simulink model "test_origin"  (R2024b)
settings: Solver=VariableStepAuto  StartTime=0.0  StopTime=2  RelTol=1e-3
values from neighbouring files (symbols this model uses):
  B = zeros(img_h, img_w)    [code_params.m]
  eye_mat = eye(3)    [code_params.m]
  K = [fx, s, cx ... (first row only)    [code_params.m]
  mesh_data =     [triangle_mesh_bus.mat]
  texture_map = zeros(texture_resol,texture_resol)    [code_params.m]
undefined symbols (not defined in the file or in its folder): camera0, duration, light_model, light_source, link, link_name, model_name, world_pose
libraries: robotgazebolib x10, robotcorelib x2
(part 1 of 2)
settings Model: Creator=seunghyunpyo  LastModifiedBy=seunghyunpyo

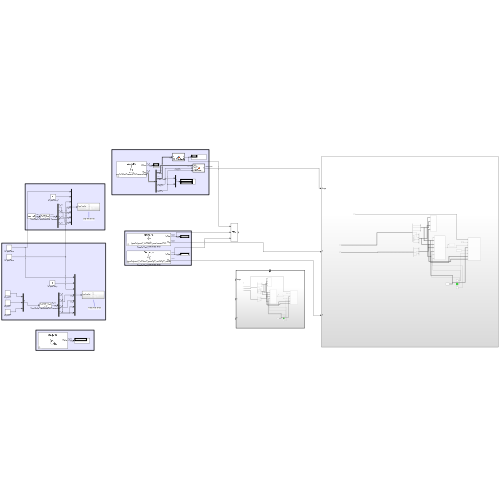
[thumbnail: Simulink's stored preview of the top-level diagram]
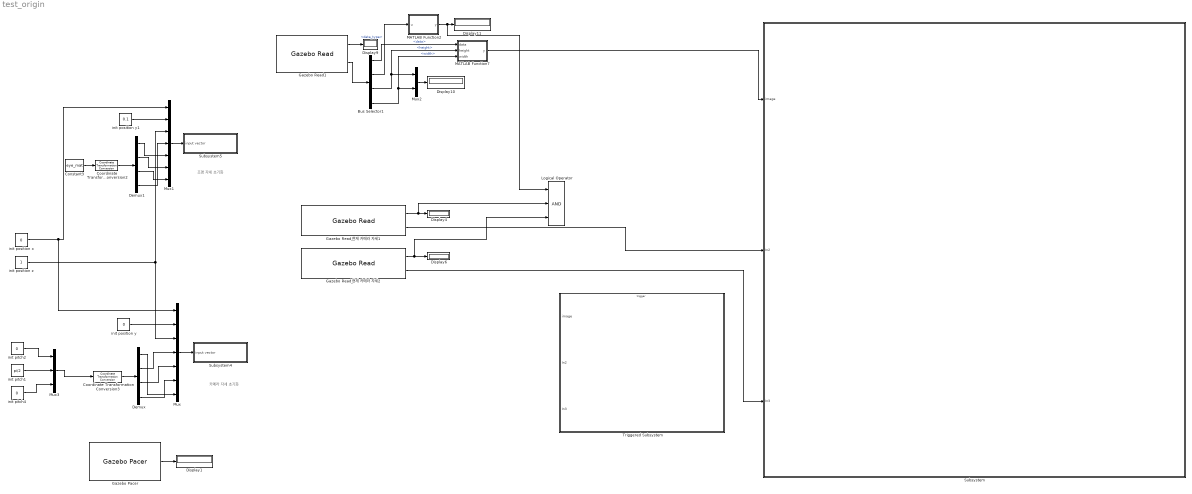
== system test_origin ==
  note: 카메라 자세 초기화
  note: 조명 자세 초기화
  Bus Selector1 : BusSelector  OutputSignals=data,data_type,height,width
  Constant3 : Constant  Value=eye_mat
  Coordinate Transformation Conversion2 : robotcorelib/Coordinate Transformation Conversion  InputRepresentation=Rotation Matrix  InputEulerSequence=ZYX  ShowTrVecInputPort=on  OutputRepresentation=Quaternion  OutputEulerSequence=XYZ  ShowTrVecOutputPort=on  SimulateUsing=Interpreted execution
  Coordinate Transformation Conversion3 : robotcorelib/Coordinate Transformation Conversion  InputRepresentation=Euler Angles  InputEulerSequence=XYZ  ShowTrVecInputPort=on  OutputRepresentation=Quaternion  OutputEulerSequence=XYZ  ShowTrVecOutputPort=on  SimulateUsing=Interpreted execution
  Demux : Demux
  Demux1 : Demux
  Display{1,4,6,9..11} (6 alike) : Display
  Gazebo Pacer : robotgazebolib/Gazebo Pacer  ResetBehavior=Reset Gazebo simulation time  SampleTime=0.01
  Gazebo Read1 : robotgazebolib/Gazebo Read  topicSource=From Gazebo  topic=/gazebo/default/camera0/link/camera/image  messageType=gazebo_msgs/Image  sampleTime=0.01  fixedAxisBusStatus=off  jointAxisCount=2
  Gazebo Read_현재 카메라 자세1 : robotgazebolib/Gazebo Read  topicSource=From Gazebo  topic=/gazebo/ground_truth/world_pose/camera0/link  messageType=gazebo_msgs/Pose  sampleTime=0.01  fixedAxisBusStatus=off  jointAxisCount=2
  Gazebo Read_현재 카메라 자세2 : robotgazebolib/Gazebo Read  topicSource=From Gazebo  topic=/gazebo/ground_truth/world_pose/light_model/light_source  messageType=gazebo_msgs/Pose  sampleTime=0.01  fixedAxisBusStatus=off  jointAxisCount=2
  Logical Operator : Logic  Inputs=3  AllPortsSameDT=off  OutDataTypeStr=boolean
  MATLAB Function2 : MATLAB Function  TreatAsAtomicUnit=on
  MATLAB Function7 : MATLAB Function  TreatAsAtomicUnit=on
  Mux : Mux  Inputs=7
  Mux1 : Mux  Inputs=7
  Mux2 : Mux  Inputs=2
  Mux3 : Mux  Inputs=3
  Subsystem : Subsystem
  Subsystem4 : Subsystem
  Subsystem5 : Subsystem
  Triggered Subsystem : Subsystem  TreatAsAtomicUnit=on
  init pitch1 : Constant  Value=pi/2
  init pitch2 : Constant  Value=0
  init pitch4 : Constant  Value=0
  init position x : Constant  Value=0
  init position y : Constant  Value=0
  init position y1 : Constant  Value=0.1
  init position z : Constant
  wires:
  Coordinate Transformation Conversion3/1 -> Demux/1
  Demux1/3 -> Mux1/7
  Mux3/1 -> Coordinate Transformation Conversion3/1
  Demux/1 -> Mux/7
  init pitch4/1 -> Mux3/3
  init pitch2/1 -> Mux3/1
  Mux/1 -> Subsystem4/1(input vector)
  Gazebo Read1/2 -> Bus Selector1/1
  Mux2/1 -> Display10/1
  Constant3/1 -> Coordinate Transformation Conversion2/1
  init position y1/1 -> Mux1/2
  Demux/4 -> Mux/6
  Demux/3 -> Mux/5
  init position y/1 -> Mux/2
  Gazebo Pacer/1 -> Display1/1
  init position z/1 -> Mux/3, Mux1/3
  Demux/2 -> Mux/4
  init position x/1 -> Mux/1, Mux1/1
  MATLAB Function2/1(y) -> Logical Operator/1, Display11/1
  Bus Selector1/4 -> MATLAB Function7/3(width), Mux2/2  "<width>"
  Bus Selector1/2 -> MATLAB Function2/1(u)  "<data_type>"
  init pitch1/1 -> Mux3/2
  Gazebo Read1/1 -> Display9/1
  Demux1/1 -> Mux1/5
  Bus Selector1/3 -> MATLAB Function7/2(height), Mux2/1  "<height>"
  Mux1/1 -> Subsystem5/1(input vector)
  Demux1/4 -> Mux1/4
  Demux1/2 -> Mux1/6
  Bus Selector1/1 -> MATLAB Function7/1(data)  "<data>"
  Coordinate Transformation Conversion2/1 -> Demux1/1
  Gazebo Read_현재 카메라 자세2/1 -> Logical Operator/3, Display6/1
  Gazebo Read_현재 카메라 자세1/1 -> Logical Operator/2, Display4/1
  MATLAB Function7/1(y) -> Subsystem/1(image)
  Gazebo Read_현재 카메라 자세1/2 -> Subsystem/2(In2)
  Gazebo Read_현재 카메라 자세2/2 -> Subsystem/3(In3)

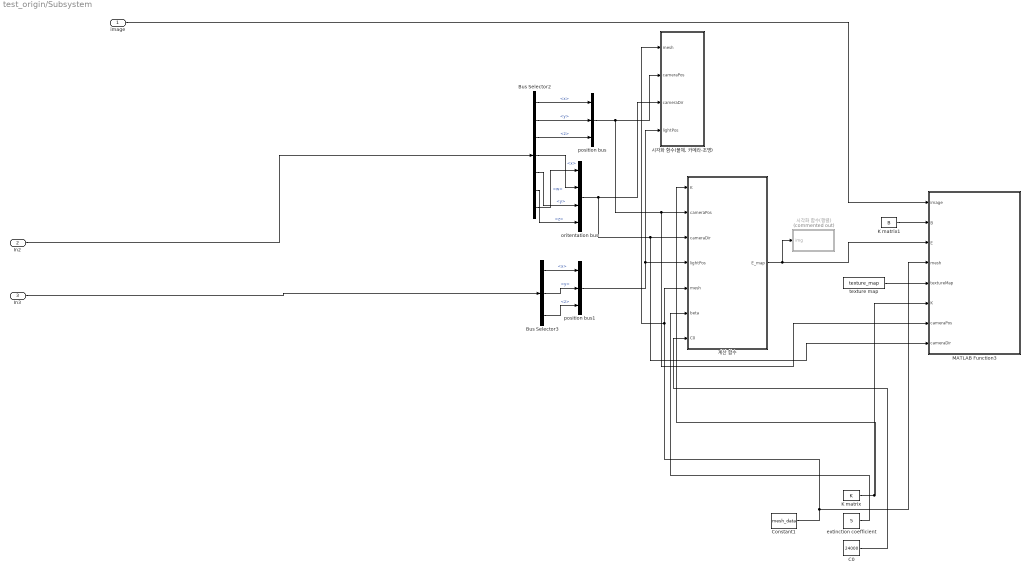
== system test_origin/Subsystem ==
  image : Inport
  In2 : Inport  Port=2
  In3 : Inport  Port=3
  Bus Selector2 : BusSelector  OutputSignals=position.x,position.y,position.z,orientation.x,orientation.y,orientation.z,orientation.w
  Bus Selector3 : BusSelector  OutputSignals=position.x,position.y,position.z
  C0 : Constant  Value=24000
  Constant1 : Constant  Value=mesh_data  OutDataTypeStr=Bus: slBus1
  K matrix : Constant  Value=K
  K matrix1 : Constant  Value=B
  MATLAB Function3 : MATLAB Function  TreatAsAtomicUnit=on
  extinction coefficient : Constant  Value=5
  oritentation bus : BusCreator  Inputs=4
  position bus : BusCreator  Inputs=3
  position bus1 : BusCreator  Inputs=3
  texture map : Constant  Value=texture_map
  계산 함수 : MATLAB Function  TreatAsAtomicUnit=on
  "시각화 함수(물체, 카메라-조명)" : MATLAB Function  TreatAsAtomicUnit=on
  시각화 함수(행렬) : MATLAB Function  Commented=on  TreatAsAtomicUnit=on
  wires:
  In3/1 -> Bus Selector3/1
  image/1 -> MATLAB Function3/1(image)
  Bus Selector2/6 -> oritentation bus/4  "<z>"
  In2/1 -> Bus Selector2/1
  Bus Selector2/4 -> oritentation bus/2  "<x>"
  oritentation bus/1 -> MATLAB Function3/8(cameraDir), 계산 함수/3(cameraDir), "시각화 함수(물체, 카메라-조명)"/3(cameraDir)
  position bus/1 -> MATLAB Function3/7(cameraPos), 계산 함수/2(cameraPos), "시각화 함수(물체, 카메라-조명)"/2(cameraPos)
  Bus Selector3/1 -> position bus1/1  "<x>"
  Bus Selector2/1 -> position bus/1  "<x>"
  Bus Selector2/3 -> position bus/3  "<z>"
  Bus Selector3/2 -> position bus1/2  "<y>"
  Bus Selector3/3 -> position bus1/3  "<z>"
  Bus Selector2/2 -> position bus/2  "<y>"
  position bus1/1 -> 계산 함수/4(lightPos), "시각화 함수(물체, 카메라-조명)"/4(lightPos)
  C0/1 -> 계산 함수/7(C0)
  Bus Selector2/5 -> oritentation bus/3  "<y>"
  texture map/1 -> MATLAB Function3/5(textureMap)
  Bus Selector2/7 -> oritentation bus/1  "<w>"
  K matrix1/1 -> MATLAB Function3/2(B)
  Constant1/1 -> MATLAB Function3/4(mesh), "시각화 함수(물체, 카메라-조명)"/1(mesh), 계산 함수/5(mesh)
  K matrix/1 -> MATLAB Function3/6(K), 계산 함수/1(K)
  계산 함수/1(E_map) -> 시각화 함수(행렬)/1(img), MATLAB Function3/3(E)
  extinction coefficient/1 -> 계산 함수/6(beta)

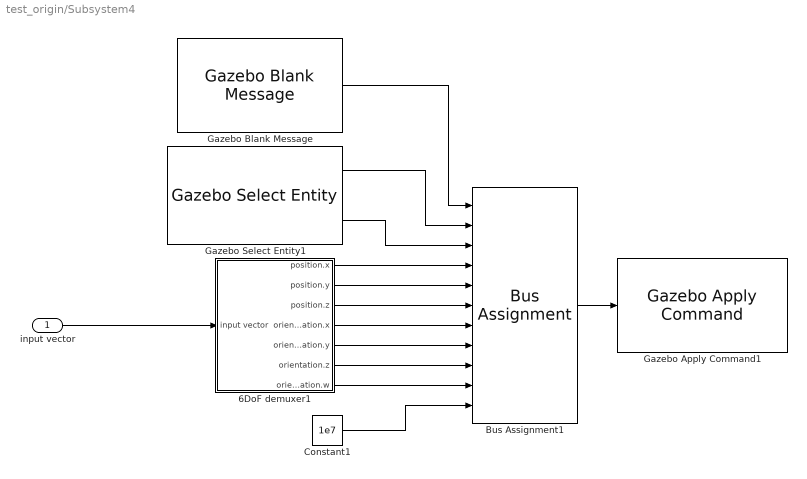
== system test_origin/Subsystem4 ==
  input vector : Inport
  6DoF demuxer1 : Subsystem
  Bus Assignment1 : BusAssignment  AssignedSignals=model_name,link_name,world_pose.position.x,world_pose.position.y,world_pose.position.z,world_pose.orientation.x,world_pose.orientation.y,world_pose.orientation.z,world_pose.orientation.w,duration.nano_seconds
  Constant1 : Constant  Value=1e7
  Gazebo Apply Command1 : robotgazebolib/Gazebo Apply Command  cmdType=SetLinkWorldPose  sampleTime=0.01
  Gazebo Blank Message : robotgazebolib/Gazebo Blank Message  msgType=SetLinkWorldPose  sampleTime=0.01  busName='Gazebo_SL_Bus_gazebo_msgs_SetLinkWorldPose'
  Gazebo Select Entity1 : robotgazebolib/Gazebo Select Entity  modelElemName=camera0/link  outputArraySize=128  OutputLabel=Link  SelectType=Link
  wires:
  Constant1/1 -> Bus Assignment1/11
  6DoF demuxer1/1(position.x) -> Bus Assignment1/4
  6DoF demuxer1/2(position.y) -> Bus Assignment1/5
  input vector/1 -> 6DoF demuxer1/1(input vector)
  Bus Assignment1/1 -> Gazebo Apply Command1/1
  Gazebo Blank Message/1 -> Bus Assignment1/1
  6DoF demuxer1/6(orientation.z) -> Bus Assignment1/9
  6DoF demuxer1/3(position.z) -> Bus Assignment1/6
  6DoF demuxer1/5(orientation.y) -> Bus Assignment1/8
  6DoF demuxer1/4(orientation.x) -> Bus Assignment1/7
  Gazebo Select Entity1/2 -> Bus Assignment1/3
  Gazebo Select Entity1/1 -> Bus Assignment1/2
  6DoF demuxer1/7(orientation.w) -> Bus Assignment1/10

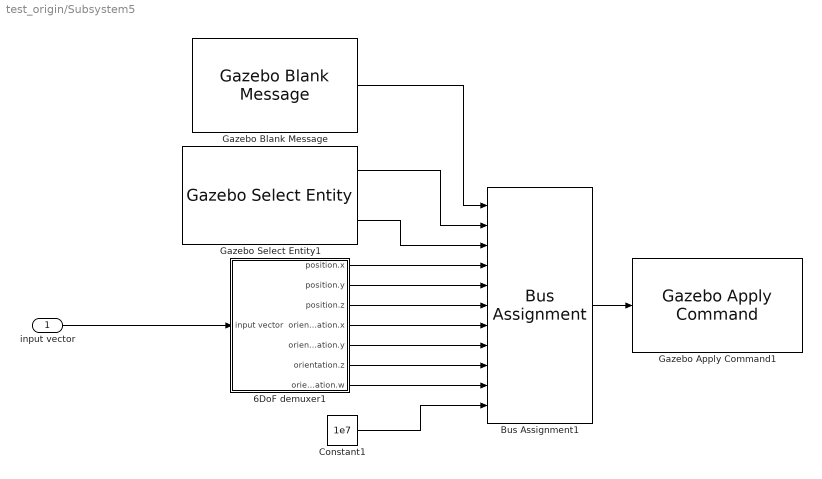
== system test_origin/Subsystem5 ==
  input vector : Inport
  6DoF demuxer1 : Subsystem
  Bus Assignment1 : BusAssignment  AssignedSignals=model_name,link_name,world_pose.position.x,world_pose.position.y,world_pose.position.z,world_pose.orientation.x,world_pose.orientation.y,world_pose.orientation.z,world_pose.orientation.w,duration.nano_seconds
  Constant1 : Constant  Value=1e7
  Gazebo Apply Command1 : robotgazebolib/Gazebo Apply Command  cmdType=SetLinkWorldPose  sampleTime=0.01
  Gazebo Blank Message : robotgazebolib/Gazebo Blank Message  msgType=SetLinkWorldPose  sampleTime=0.01  busName='Gazebo_SL_Bus_gazebo_msgs_SetLinkWorldPose'
  Gazebo Select Entity1 : robotgazebolib/Gazebo Select Entity  modelElemName=light_model/light_source  outputArraySize=128  OutputLabel=Link  SelectType=Link
  wires:
  6DoF demuxer1/7(orientation.w) -> Bus Assignment1/10
  Gazebo Select Entity1/1 -> Bus Assignment1/2
  Gazebo Select Entity1/2 -> Bus Assignment1/3
  6DoF demuxer1/4(orientation.x) -> Bus Assignment1/7
  6DoF demuxer1/5(orientation.y) -> Bus Assignment1/8
  6DoF demuxer1/3(position.z) -> Bus Assignment1/6
  6DoF demuxer1/6(orientation.z) -> Bus Assignment1/9
  Gazebo Blank Message/1 -> Bus Assignment1/1
  Bus Assignment1/1 -> Gazebo Apply Command1/1
  6DoF demuxer1/2(position.y) -> Bus Assignment1/5
  6DoF demuxer1/1(position.x) -> Bus Assignment1/4
  Constant1/1 -> Bus Assignment1/11
  input vector/1 -> 6DoF demuxer1/1(input vector)

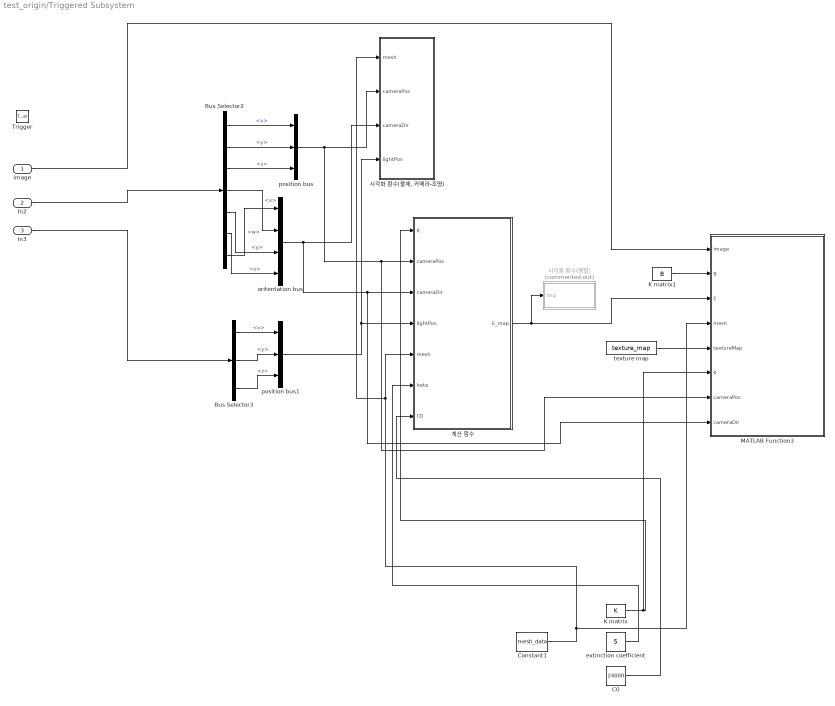
== system test_origin/Triggered Subsystem ==
  image : Inport
  In2 : Inport  Port=2
  In3 : Inport  Port=3
  Trigger : TriggerPort  VariantControl=(inherit)
  Bus Selector2 : BusSelector  OutputSignals=position.x,position.y,position.z,orientation.x,orientation.y,orientation.z,orientation.w
  Bus Selector3 : BusSelector  OutputSignals=position.x,position.y,position.z
  C0 : Constant  Value=24000
  Constant1 : Constant  Value=mesh_data  OutDataTypeStr=Bus: slBus1
  K matrix : Constant  Value=K
  K matrix1 : Constant  Value=B
  MATLAB Function3 : MATLAB Function  TreatAsAtomicUnit=on
  extinction coefficient : Constant  Value=5
  oritentation bus : BusCreator  Inputs=4
  position bus : BusCreator  Inputs=3
  position bus1 : BusCreator  Inputs=3
  texture map : Constant  Value=texture_map
  계산 함수 : MATLAB Function  TreatAsAtomicUnit=on
  "시각화 함수(물체, 카메라-조명)" : MATLAB Function  TreatAsAtomicUnit=on
  시각화 함수(행렬) : MATLAB Function  Commented=on  TreatAsAtomicUnit=on
  wires:
  image/1 -> MATLAB Function3/1(image)
  Bus Selector2/6 -> oritentation bus/4  "<z>"
  In3/1 -> Bus Selector3/1
  In2/1 -> Bus Selector2/1
  계산 함수/1(E_map) -> 시각화 함수(행렬)/1(img), MATLAB Function3/3(E)
  K matrix/1 -> MATLAB Function3/6(K), 계산 함수/1(K)
  Constant1/1 -> MATLAB Function3/4(mesh), "시각화 함수(물체, 카메라-조명)"/1(mesh), 계산 함수/5(mesh)
  position bus1/1 -> 계산 함수/4(lightPos), "시각화 함수(물체, 카메라-조명)"/4(lightPos)
  Bus Selector2/4 -> oritentation bus/2  "<x>"
  texture map/1 -> MATLAB Function3/5(textureMap)
  extinction coefficient/1 -> 계산 함수/6(beta)
  position bus/1 -> MATLAB Function3/7(cameraPos), 계산 함수/2(cameraPos), "시각화 함수(물체, 카메라-조명)"/2(cameraPos)
  Bus Selector3/3 -> position bus1/3  "<z>"
  Bus Selector2/2 -> position bus/2  "<y>"
  C0/1 -> 계산 함수/7(C0)
  Bus Selector3/2 -> position bus1/2  "<y>"
  oritentation bus/1 -> MATLAB Function3/8(cameraDir), 계산 함수/3(cameraDir), "시각화 함수(물체, 카메라-조명)"/3(cameraDir)
  Bus Selector2/3 -> position bus/3  "<z>"
  Bus Selector3/1 -> position bus1/1  "<x>"
  K matrix1/1 -> MATLAB Function3/2(B)
  Bus Selector2/5 -> oritentation bus/3  "<y>"
  Bus Selector2/7 -> oritentation bus/1  "<w>"
  Bus Selector2/1 -> position bus/1  "<x>"

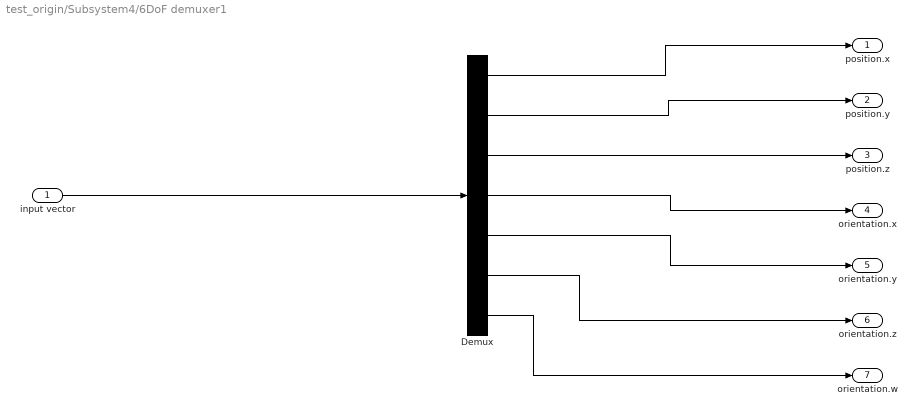
== system test_origin/Subsystem4/6DoF demuxer1 ==
  input vector : Inport
  Demux : Demux  Outputs=7
  position.x : Outport
  position.y : Outport  Port=2
  position.z : Outport  Port=3
  orientation.x : Outport  Port=4
  orientation.y : Outport  Port=5
  orientation.z : Outport  Port=6
  orientation.w : Outport  Port=7
  wires:
  input vector/1 -> Demux/1
  Demux/1 -> position.x/1
  Demux/2 -> position.y/1
  Demux/3 -> position.z/1
  Demux/4 -> orientation.x/1
  Demux/5 -> orientation.y/1
  Demux/6 -> orientation.z/1
  Demux/7 -> orientation.w/1

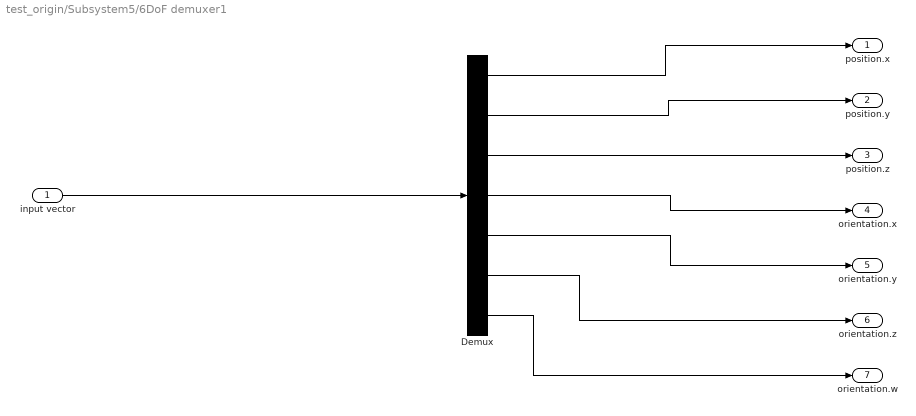
== system test_origin/Subsystem5/6DoF demuxer1 ==
  input vector : Inport
  Demux : Demux  Outputs=7
  position.x : Outport
  position.y : Outport  Port=2
  position.z : Outport  Port=3
  orientation.x : Outport  Port=4
  orientation.y : Outport  Port=5
  orientation.z : Outport  Port=6
  orientation.w : Outport  Port=7
  wires:
  Demux/7 -> orientation.w/1
  Demux/6 -> orientation.z/1
  Demux/5 -> orientation.y/1
  Demux/4 -> orientation.x/1
  Demux/3 -> position.z/1
  Demux/2 -> position.y/1
  Demux/1 -> position.x/1
  input vector/1 -> Demux/1

== matlab function test_origin/MATLAB Function7 ==
  data: data input; height input; width input; y output [..255]
function y  = plotImage(data, height, width)

coder.extrinsic('imshow');
coder.extrinsic('helperPlotImage');

persistent h

if isempty(h)
    h = newplot(figure());
end


y = zeros(height, width, 3, 'uint8');
if ~isempty(data) && ~isscalar(data)
    y(:) = helperPlotImage(data, height, width);
end
imshow(y, 'Parent', h);

== matlab function test_origin/Subsystem/시각화 함수(물체, 카메라-조명) ==
  data: mesh input; cameraPos input; cameraDir input; lightPos input
function viz_scene(mesh, cameraPos, cameraDir, lightPos)

    persistent figHandle; % Figure 핸들을 저장할 persistent 변수

    if isempty(figHandle)
        % Figure가 없으면 (처음 실행) figHandle 초기화
        figHandle = figure;
        set(figHandle, 'Name', 'Scene Visualization'); % (선택 사항) 창 제목 설정
    elseif ~ishandle(figHandle) || ~strcmp(get(figHandle, 'Type'), 'figure')
        % Figure 핸들이 유효하지 않으면 (Figure가 닫힌 경우)
        figHandle = figure; % 새 Figure 생성
        set(figHandle, 'Name', 'Scene Visualization');
    end
    
    figure(figHandle); % 해당 Figure를 활성화
    clf;    % Figure 내용 clear  % clf(figHandle) 대신 clf 사용

    faces_vertex = mesh.faces.v;
    vertices = mesh.vertices;
    quat_link_world = quaternion(cameraDir(1), cameraDir(2), cameraDir(3), cameraDir(4));
    R_w2link = rotmat(quat_link_world, 'frame');         % 월드 -> 링크 좌표계 회전
    R_link2cam =[0 -1 0; 0 0 -1; 1 0 0];                % 링크 좌표계 -> 카메라 좌표계 회전


    % 1. 메쉬 그리기
    subplot(1, 2, 1); % 이 부분은 그대로 유지
    trisurf(faces_vertex, vertices(:,1), vertices(:,2), vertices(:,3), 'FaceColor', 'cyan', 'EdgeColor', 'k');
    hold on;
    % Face 중앙에 Face 번호 표시
    for i = 1:int32(size(faces_vertex, 1))
        % 현재 Face의 정점 3개 가져오기
        face_vertices = vertices(faces_vertex(i, :), :);

        % Face의 중심 좌표 계산
        face_center = mean(face_vertices, 1);

        % Face의 중앙에 번호 표시
        text(face_center(1), face_center(2), face_center(3), sprintf('%d',i), ...
            'FontSize', 12, 'FontWeight', 'bold', 'Color', 'r');
    end

    % 2. 카메라 위치 및 방향 (월드 좌표계)
    cameraPos_world = cameraPos; % 월드 좌표계에서의 카메라 위치
    R_world_to_cam = R_link2cam * R_w2link; % 카메라 방향 변환 행렬
    % 카메라 X축 (빨강)
    quiver3(cameraPos_world(1), cameraPos_world(2), cameraPos_world(3), ...
        R_world_to_cam(1,1), R_world_to_cam(2,1), R_world_to_cam(3,1), 0.3, 'r', 'LineWidth', 2, 'MaxHeadSize', 0.5);
    % 카메라 Y축 (초록)
    quiver3(cameraPos_world(1), cameraPos_world(2), cameraPos_world(3), ...
        R_world_to_cam(1,2), R_world_to_cam(2,2), R_world_to_cam(3,2), 0.3, 'g', 'LineWidth', 2, 'MaxHeadSize', 0.5);
    % 카메라 Z축 (파랑)
    quiver3(cameraPos_world(1), cameraPos_world(2), cameraPos_world(3), ...
        R_world_to_cam(1,3), R_world_to_cam(2,3), R_world_to_cam(3,3), 0.3, 'b', 'LineWidth', 2, 'MaxHeadSize', 0.5);

    % 카메라 위치 (빨간색 점)
    plot3(cameraPos_world(1), cameraPos_world(2), cameraPos_world(3), 'ro', 'MarkerSize', 8, 'MarkerFaceColor', 'r');
    % 3. 광원 위치
    plot3(lightPos(1), lightPos(2), lightPos(3), 'yo', 'MarkerSize', 10, 'MarkerFaceColor', 'y'); % 노란색 점
    % 축 및 레이블
    xlabel('X (World)');
    ylabel('Y (World)');
    zlabel('Z (World)');
    title('World Coordinate System (Mesh, Camera, Light)');
    axis equal;
    grid on;
    view(3);
    hold off;
end

== matlab function test_origin/Subsystem/시각화 함수(행렬) ==
  data: img input
function viz_mat(img)
    figure;
    imagesc(img);
    colorbar;
    title('E\_map (Scattering Lighting)');
    xlabel('Pixel X');
    ylabel('Pixel Y');
    axis image; % x, y 축 비율을 데이터에 맞게
end

== matlab function test_origin/Subsystem/계산 함수 ==
  data: K input; cameraPos input; cameraDir input; lightPos input; mesh input; beta input; C0 input; E_map output
function E_map = computeScatteringLighting(K, cameraPos, cameraDir, lightPos, mesh, beta, C0)
    % 입력:
    %   K: 3x3 Intrinsic Matrix (카메라 내부 파라미터 행렬)
    %   R_link: 3x3 Rotation Matrix (월드 좌표계 -> 링크 좌표계 회전 행렬)
    %   T: 3x1 Translation Vector (월드 좌표계 -> 링크 좌표계 이동 벡터)
    %   lightPos: 1x3 광원 위치 (월드 좌표계)
    %   mesh: 메쉬 데이터 (구조체)
    %       mesh.v:  정점(Vertices) 좌표 (Nx3 행렬, N: 정점 개수)
    %       mesh.f.v: 면(Faces)을 구성하는 정점 인덱스 (Mx3 행렬, M: 면 개수)
    %       mesh.f.vn: 면의 법선 벡터 (Mx3 행렬)
    %   beta: 감쇠 계수 (Attenuation Coefficient)
    %   C0: 광원의 초기 강도 (Initial Light Intensity)
    imageHeight = 480;
    imageWidth = 640;

    % 출력:
    %   E_map: imageHeight x imageWidth 크기의 2D 이미지. 각 픽셀은 해당 위치에 도달하는 빛의 에너지(세기)를 나타냄.

    % 1. 메쉬 데이터 가져오기
    vertices = mesh.vertices;      % 정점 좌표
    faces_vertex = mesh.faces.v; % 면을 구성하는 정점 인덱스
    normals = mesh.faces.vn;    % 면의 법선 벡터

    % 2. 출력 맵 초기화
    E_map = zeros(imageHeight, imageWidth); % 출력 이미지를 0으로 초기화
    numFaces = size(faces_vertex, 1);     % 면의 개수

    % 3. 월드 좌표계 -> 카메라 좌표계 변환 행렬 계산
    T_link = cameraPos; % 나중에 전치 주의!!

    quat_link_world = quaternion(cameraDir(1), cameraDir(2), cameraDir(3), cameraDir(4));
    R_w2link = rotmat(quat_link_world, 'frame')         % 월드 -> 링크 좌표계 회전
    R_link2cam =[0 -1 0; 0 0 -1; 1 0 0];                % 링크 좌표계 -> 카메라 좌표계 회전 
    
    Proj_w2link = [R_w2link, -R_w2link*T_link; 0,0,0,1];        % 동차 변환 행렬 (월드 -> 링크)
    Proj_link2Cam = [R_link2cam, zeros(3,1); zeros(1,3), 1];    % 동차 변환 행렬 (링크 -> 카메라)
    Proj_w2cam = Proj_link2Cam * Proj_w2link;                   % 동차 변환 행렬 (월드 -> 카메라)

    % 4. 광원 위치를 카메라 좌표계로 변환 (동차 좌표계 사용)
    lightPos_hom = [lightPos; 1]; % 광원 위치를 동차 좌표로
    lightPosCam_hom = Proj_w2cam * lightPos_hom;
    lightPosCam = lightPosCam_hom(1:3); % 다시 3차원 좌표로
    
   % 5. 각 면에 대해 반복
    for i = 1:numFaces
        % 5.1. 면의 세 정점 좌표 (월드 좌표계)
        v1 = vertices(faces_vertex(i, 1), :); % 첫 번째 정점
        v2 = vertices(faces_vertex(i, 2), :); % 두 번째 정점
        v3 = vertices(faces_vertex(i, 3), :); % 세 번째 정점

        % 5.2. 면 중심 (월드 좌표계)
        faceCenter = (v1 + v2 + v3) / 3;

        % 5.3. 면의 법선 벡터 (월드 좌표계, 정규화)
        normal = normals(i, :);
        normal = normal / norm(normal);

        % 5.4. 카메라 좌표계로 변환 (동차 좌표계 사용)
        faceCenter_hom = [faceCenter, 1]';
        faceCenterCam_hom = Proj_w2cam * faceCenter_hom;
        faceCenterCam = faceCenterCam_hom(1:3);

        v1_hom = [v1, 1]';
        v1_cam_hom = Proj_w2cam * v1_hom;
        v1_cam = v1_cam_hom(1:3);

        v2_hom = [v2, 1]';
        v2_cam_hom = Proj_w2cam * v2_hom;
        v2_cam = v2_cam_hom(1:3);

        v3_hom = [v3, 1]';
        v3_cam_hom = Proj_w2cam * v3_hom;
        v3_cam = v3_cam_hom(1:3);

        normal_hom = [normal, 0]'; % 방향 벡터는 마지막 요소가 0
        normalCam_hom = Proj_w2cam * normal_hom;
        normalCam = normalCam_hom(1:3);



        % 5.5. 광원 방향 (카메라 좌표계)
        lightDir = lightPosCam - faceCenterCam; % 면 중심 -> 광원
        lLS = norm(lightDir);              % 광원과 면 중심 사이의 거리
        lightDir = lightDir / lLS;           % 정규화

        % 5.6. Lambertian 반사 계수
        diffuseFactor = max(0, dot(normalCam, lightDir)); % (0 ~ 1)

        % 5.7. 직접광 (Ds) 계산
        Ds = (C0 * exp(-beta * lLS)) / (lLS^2);

        % 5.8. 산란 지점 (z) 계산 (카메라 좌표계)
        epsilon = 0.01; % 작은 값 (면에서 약간 떨어진 거리)
        z = faceCenterCam + epsilon * normalCam; % 면 중심에서 법선 방향으로

        % 5.9. 거리 계산 (카메라 좌표계)
        lLZ = norm(lightPosCam - z);     % 광원 -> 산란 지점
        lSZ = norm(z - faceCenterCam);   % 산란 지점 -> 면 중심
        lSC = norm(faceCenterCam);       % 면 중심 -> 카메라

        % 5.10. 산란광 (As) 계산
        As = (C0 * exp(-beta * (lLZ + lSZ))) / ((lLZ + lSZ)^2);

        % 5.11. 초기 조도, 최종 조도
        Es_initial = Ds + As;            % 직접광 + 산란광
        Es = Es_initial * exp(-beta * lSC); % 최종 감쇠

        % 5.12. 각 정점을 2D 이미지 좌표로 투영 (카메라 내부 파라미터 K 사용)
        v1_proj_hom = K * v1_cam;
        v1_proj = round(v1_proj_hom(1:2) / v1_proj_hom(3)); % 2D 픽셀 좌표

        v2_proj_hom = K * v2_cam;
        v2_proj = round(v2_proj_hom(1:2) / v2_proj_hom(3));

        v3_proj_hom = K * v3_cam;
        v3_proj = round(v3_proj_hom(1:2) / v3_proj_hom(3));


        % 5.13. 삼각형 래스터화 (Bresenham's Algorithm 기반)
        pixels = [];

        % 삼각형의 세 변을 따라 픽셀 좌표 생성
        pixels = [pixels; bresenham(v1_proj(1), v1_proj(2), v2_proj(1), v2_proj(2))];
        pixels = [pixels; bresenham(v2_proj(1), v2_proj(2), v3_proj(1), v3_proj(2))];
        pixels = [pixels; bresenham(v3_proj(1), v3_proj(2), v1_proj(1), v1_proj(2))];

        % 5.14. 삼각형 내부 픽셀에 대해 반복
        for p = 1:size(pixels, 1)
             x = pixels(p, 1); % 픽셀 x 좌표
             y = pixels(p, 2); % 픽셀 y 좌표

             % 픽셀이 이미지 범위 내에 있는지 확인
            if x < 1 || x > imageWidth || y < 1 || y > imageHeight
                continue;
            end

            % Barycentric Coordinates 계산
            [alpha, beta, gamma] = barycentric(x, y, v1_proj, v2_proj, v3_proj);

            if alpha >= 0 && beta >= 0 && gamma >= 0
                % 5.15. 픽셀 (x, y)에 E_s * diffuseFactor 값을 할당
                E_map(y, x) = Es * diffuseFactor;
            end
        end
    end % for i
end % function

% Bresenham's line algorithm 함수
function points = bresenham(x1, y1, x2, y2)
    % 입력: 두 점 (x1, y1), (x2, y2)
    % 출력: 두 점을 잇는 직선 상의 픽셀 좌표 (정수)

    points = [];
    dx = abs(x2 - x1);
    dy = abs(y2 - y1);
    sx = sign(x2 - x1);
    sy = sign(y2 - y1);
    err = dx - dy;

    x = x1;
    y = y1;

    while true
        points = [points; x, y];

        if x == x2 && y == y2
            break;
        end

        e2 = 2 * err;
        if e2 > -dy
            err = err - dy;
            x = x + sx;
        end
        if e2 < dx
            err = err + dx;
            y = y + sy;
        end
    end
end

% Barycentric coordinates 계산 함수
function [alpha, beta, gamma] = barycentric(x, y, v1, v2, v3)
    % 입력:
    %   x, y: 픽셀 좌표
    %   v1, v2, v3: 삼각형의 세 꼭지점 좌표 (2D)
    % 출력:
    %    alpha, beta, gamma: Barycentric Coordinates

    % 삼각형 면적 계산 (두 벡터의 외적)
    area = 0.5 * (-v2(2) * v3(1) + v1(2) * (-v2(1) + v3(1)) + v1(1) * (v2(2) - v3(2)) + v2(1) * v3(2));

    % 각 꼭지점에 대한 가중치 계산
    alpha = 0.5 * (-v2(2) * v3(1) + y * (-v2(1) + v3(1)) + x * (v2(2) - v3(2)) + v2(1) * v3(2)) / area;
    beta  = 0.5 * ( v1(2) * v3(1) - y * v3(1) + x * (-v1(2) + v3(2)) - v1(1) * v3(2)              ) / area;
    gamma = 0.5 * (-v1(2) * v2(1) + v1(2) * x + v2(2) * (-x + v1(1)) + y * (v2(1) - v1(1))) / area;

end

== matlab function test_origin/Triggered Subsystem/MATLAB Function3 ==
  data: image input; B input; E input; mesh input; textureMap input; K input; cameraPos input; cameraDir input
function processReflectance(image, B, E, mesh, textureMap, K, cameraPos, cameraDir)

    image = double(image);
    B = double(B);
    E = double(E);
    textureMap = double(textureMap);
    texture_size = size(textureMap,1);
    mesh.uv_coords = mesh.uv_coords * texture_size; % 원래 uv_coords는 정규화되어 있기에 텍스처 맵 크기만큼 곱해줌

    % 이미지<->텍스처 맵 변환 위한 준비
    [set_idx, set_img_patch, set_uv_patch] = get_img_text_coords(K, cameraPos, cameraDir, mesh);
    T_affines = calculate_affine_matrices(set_img_patch, set_uv_patch);
    set_idx
    
   
    % 반사율 계산
    epsilon = 1e-6;
    rho = (image - B) ./ (E + epsilon);
    % imshow(rho, []);
    
    % 분산 계산
    sigma_squared = computeVariance(rho, B, E);
    % imshow(sigma_squared, []);

    % 워프된 분산 획득 - 텍스처 맵 크기
    sigma_texture = dispersed_warping_and_patch_based_correction(sigma_squared, T_affines, set_img_patch, texture_size, mesh, 10);
    % imshow(sigma_texture, []);

    % 반사율 워핑 - 텍스처 맵 크기
    warpedRho = warp_texture_map(rho, T_affines, set_img_patch, texture_size);
    % imshow(warpedRho, []);

    % MLE 계산 - 텍스처 맵 크기
    rho_ML = computeMLE(warpedRho, sigma_texture, textureMap);
    % imshow(rho_ML, []);

    % 텍스처 맵 갱신
    textureMap = updateTextureMap(textureMap, warpedRho, sigma_texture);
    
    % 분산 갱신
    variance = sigma_texture;
end



function sigma_squared = computeVariance(rho, B, E)
    % 분산 계산 (식 32)
    % 입력: rho - 반사율 값, B - 산란광, E - 조명 강도
    % 출력: sigma_squared - 픽셀 기반 분산
    sigma_RN = 1e-3; % Readout noise
    sigma_squared = (rho .* E + B + sigma_RN^2) ./ (E.^2);
end

function sigma_texture = dispersed_warping_and_patch_based_correction(sigma_squared, T_affines, set_img_patch, texture_size, mesh, eta)
    % 분산 워핑 및 공간 패치 기반 보정

    % 입력 인자:
    %   sigma_squared: 카메라 좌표계의 분산
    %   T_affines: 각 면의 변환 행렬 (셀 배열)
    %   set_img_patch: 각 면에 대응하는 이미지 패치 (셀 배열)
    %   texture_size: 텍스처 맵 크기
    %   mesh: 메쉬 데이터
    %   eta: 공식 34에 사용되는 파라미터 (기본값: 10)

    % 출력 인자:
    %   sigma_texture: 보정된 텍스처 좌표계의 분산

    % 1. 카메라 좌표계의 분산을 텍스처 좌표계로 워핑
    warped_sigma = warp_texture_map(sigma_squared, T_affines, set_img_patch, texture_size);

    % 2. 메쉬 기반으로 U_s (각 패치의 크기) 계산
    Us = computePatchSizes(mesh);

    % 3. 패치 크기 기반 보정 (조건에 따라 공식 33 또는 34 적용)
    sigma_texture = zeros(size(warped_sigma)); % 결과 초기화
    for i = 1:length(Us)
        if Us(i) >= 1
            % 공식 33: |U_s| >= 1
            sigma_texture(i) = (1 / Us(i)) * warped_sigma(i);
        else
            % 공식 34: |U_s| <= 1
            sigma_texture(i) = exp(eta * (1 / Us(i) - 1)) * warped_sigma(i);
        end
    end
end

function Us = computePatchSizes(mesh)
    % 메쉬에서 각 패치의 크기 계산 (UV 좌표 기반)
    % mesh: vertices, faces, UV 정보 포함
    
    % 삼각형의 면 정보와 UV 좌표 가져오기
    faces_uv = mesh.faces.vt; % 삼각형 면에 해당하는 uv상 정점 (Nx3, 각 행이 삼각형의 정점 인덱스)
    UV = mesh.uv_coords;       % UV 좌표 (Mx2, 정점별 UV 좌표)
    
    % 삼각형 면적 계산 (UV 좌표계)
    % 각 삼각형의 세 꼭짓점의 UV 좌표
    UV1 = UV(faces_uv(:,1), :); % 첫 번째 꼭짓점
    UV2 = UV(faces_uv(:,2), :); % 두 번째 꼭짓점
    UV3 = UV(faces_uv(:,3), :); % 세 번째 꼭짓점
    
    % 벡터 계산
    edge1 = UV2 - UV1; % 첫 번째 변
    edge2 = UV3 - UV1; % 두 번째 변
    
    % 삼각형 면적 계산 (벡터 외적의 크기)
    Us = 0.5 * abs(edge1(:,1) .* edge2(:,2) - edge1(:,2) .* edge2(:,1)); % |u1*v2 - u2*v1|
    
    % Us는 각 삼각형 면적의 배열로 반환됩니다
end


function rho_ML = computeMLE(rho, variance, texture_map)
    % MLE 계산 (식 17)
    % 입력: rho - 반사율 값, variance - 품질 분산
    % 출력: rho_ML - 최대우도 반사율
    % weight = 1 ./ variance;
    % rho_ML = sum(weight .* rho, 'all') / sum(weight, 'all');
    rho_ML = rho;
end

function textureMap = updateTextureMap(textureMap, warpedRho, variance)
    % 기존 텍스처 맵과 워핑된 반사율 값의 가중 평균
    w1 = 0.5; % textureMap의 가중치
    w2 = 0.5; % warpedRho의 가중치
    weight = 1 ./ variance;
    % textureMap = (w1 .* textureMap .* weight + w2 .* warpedRho .* weight) ./ (w1 + w2);
    textureMap = (w1 .* textureMap+ w2 .* warpedRho) ./ (w1 + w2);
end

function [set_idx, set_img_patch, set_uv_patch] = get_img_text_coords(K, cameraPos, cameraDir, mesh)
    % 입력되는 메쉬의 UV좌표계는 픽셀!!! 0~1 아님!!!

    % 1. 메쉬 데이터 가져오기
    vertices = mesh.vertices;      % 정점 좌표
    faces_vertex = mesh.faces.v; % 면을 구성하는 정점 인덱스

    numFaces = size(faces_vertex, 1);     % 면의 개수

    % 월드 좌표계 -> 카메라 좌표계 변환 행렬 계산
    T_link = cameraPos; % 나중에 전치 주의!!

    quat_link_world = quaternion(cameraDir(1), cameraDir(2), cameraDir(3), cameraDir(4));
    R_w2link = rotmat(quat_link_world, 'frame');         % 월드 -> 링크 좌표계 회전
    R_link2cam =[0 -1 0; 0 0 -1; 1 0 0];                % 링크 좌표계 -> 카메라 좌표계 회전 
    
    Proj_w2link = [R_w2link, -R_w2link*T_link; 0,0,0,1];        % 동차 변환 행렬 (월드 -> 링크)
    Proj_link2Cam = [R_link2cam, zeros(3,1); zeros(1,3), 1];    % 동차 변환 행렬 (링크 -> 카메라)
    Proj_w2cam = Proj_link2Cam * Proj_w2link;                   % 동차 변환 행렬 (월드 -> 카메라)
    
    set_idx = [];
    set_img_patch = {};
    set_uv_patch = {};
    
   % 각 면에 대해 반복
    for i = 1:numFaces
        %  면의 세 정점 좌표 (월드 좌표계)
        v1 = vertices(faces_vertex(i, 1), :); % 첫 번째 정점
        v2 = vertices(faces_vertex(i, 2), :); % 두 번째 정점
        v3 = vertices(faces_vertex(i, 3), :); % 세 번째 정점

        % 가시성 계산
        face_center = (v1 + v2 + v3) / 3; % 면의 중심
        normal = cross(v2 - v1, v3 - v1); % 면의 법선 벡터
        normal = normal / norm(normal);  % 단위 벡터로 정규화
        
        to_camera = face_center - T_link'; % 면 중심에서 카메라까지의 벡터
        visibility = dot(normal, to_camera);
        if  visibility <= 0
            % 이미지 좌표 계산
            v1_proj = project_to_image(K, Proj_w2cam, v1);
            v2_proj = project_to_image(K, Proj_w2cam, v2);
            v3_proj = project_to_image(K, Proj_w2cam, v3);
            img_patch = [v1_proj; v2_proj; v3_proj];
    
            % 텍스처 좌표계에서 UV 좌표 가져오기
            faces_uv = mesh.faces.vt;
            uv1 = mesh.uv_coords(faces_uv(i, 1), :); % 첫 번째 정점의 UV 좌표
            uv2 = mesh.uv_coords(faces_uv(i, 2), :); % 두 번째 정점의 UV 좌표
            uv3 = mesh.uv_coords(faces_uv(i, 3), :); % 세 번째 정점의 UV 좌표
            uv_patch = [uv1; uv2; uv3];

            % 계산한 값만 배열에 저장
            set_idx(end+1) = i;
            set_img_patch{end+1} = img_patch;
            set_uv_patch{end+1} = uv_patch;
            
        else
            continue; % 카메라에서 보이지 않는 면은 처리하지 않음
        end

    end % for i

end


function proj_coords = project_to_image(K, Proj_w2cam, v)
    v_hom = [v, 1]';
    v_cam = Proj_w2cam * v_hom;
    v_proj_hom = K * v_cam(1:3);
    proj_coords = round(v_proj_hom(1:2) / v_proj_hom(3));
    proj_coords = proj_coords';
end

function T_affines = calculate_affine_matrices(image_coords, uv_coords)
    % 면 개수
    numFaces = length(image_coords);

    % 변환 행렬 저장할 셀 배열 초기화
    T_affines = cell(numFaces, 1);

    % 각 면에 대해 변환 행렬 계산
    for i = 1:numFaces
        % 이미지 좌표계의 정점 (3x2)
        P_img = [
            image_coords{i}';   % (x, y) 좌표 (2x3로 전치)
            ones(1, 3)          % 동차 좌표
        ]; 

        % 텍스처 좌표계의 정점 (3x2)
        P_tex = [
            uv_coords{i}';      % (u, v) 좌표 (2x3로 전치)
            ones(1, 3)          % 동차 좌표
        ];

        % 변환 행렬 계산
        T_affines{i} = P_tex / P_img; % T_affine = P_tex * inv(P_img)
    end
end

function texture_map = warp_texture_map(image, T_affines, image_coords, texture_size)
    % image: 원본 이미지 (HxWx3)
    % T_affines: 각 면의 변환 행렬 (셀 배열)
    % image_coords: 이미지 좌표계 정점 (셀 배열)
    % texture_size: 텍스처 맵 크기 (예: [512, 512])
    
    % 텍스처 맵 초기화
    texture_map = zeros(texture_size, texture_size, size(image, 3));
    
    % 각 삼각형 면에 대해 반복
    for i = 1:length(T_affines)
        % 1. 이미지 좌표 정점 가져오기
        P_img = image_coords{i};

        % 2. 삼각형 영역의 경계 계산 (bounding box)
        x_min = max(ceil(min(P_img(:, 1))), 1);
        x_max = min(floor(max(P_img(:, 1))), size(image, 2));
        y_min = max(ceil(min(P_img(:, 2))), 1);
        y_max = min(floor(max(P_img(:, 2))), size(image, 1));
        
        % 3. 삼각형 영역의 모든 픽셀 좌표 생성
        [X, Y] = meshgrid(x_min:x_max, y_min:y_max);
        pixel_coords = [X(:), Y(:)];
        
        % 4. 픽셀이 삼각형 내부에 있는지 검사
        in_triangle = point_in_triangle(pixel_coords, P_img);
        pixel_coords = pixel_coords(in_triangle, :); % 삼각형 내부 픽셀만 선택
        
        % 5. 이미지 좌표 -> 텍스처 좌표 변환
        % 동차 좌표 사용
        pixel_coords_hom = [pixel_coords, ones(size(pixel_coords, 1), 1)]'; % 3xN
        tex_coords_hom = T_affines{i} * pixel_coords_hom; % 3xN
        tex_coords = bsxfun(@rdivide, tex_coords_hom(1:2, :), tex_coords_hom(3, :))'; % Nx2
        
        % 6. 텍스처 좌표를 텍스처 맵의 픽셀 단위로 변환
        tex_coords_pixel = round(tex_coords);
        tex_coords_pixel(:, 1) = max(min(tex_coords_pixel(:, 1), texture_size), 1); % x 좌표 제한
        tex_coords_pixel(:, 2) = max(min(tex_coords_pixel(:, 2), texture_size), 1); % y 좌표 제한
        
        % 7. 이미지 픽셀 값을 텍스처 맵에 복사 및 시각화
        for j = 1:size(pixel_coords, 1)
            img_x = pixel_coords(j, 1);
            img_y = pixel_coords(j, 2);
            tex_x = tex_coords_pixel(j, 1);
            tex_y = tex_coords_pixel(j, 2);
            
            val_img = image(img_y, img_x, :);
            double_img = double(val_img) / 255;
            texture_map(tex_y, tex_x, :) = double_img;
        end
    end
end

function is_inside = point_in_triangle(points, triangle)
    % points: Nx2 행렬 (x, y 좌표)
    % triangle: 3x2 행렬 (삼각형의 세 정점 좌표)
    % 결과: points가 삼각형 내부에 있는지 여부 (Nx1 논리 벡터)
    
    % 삼각형의 세 정점
    v1 = triangle(1, :);
    v2 = triangle(2, :);
    v3 = triangle(3, :);
    
    % 각 변의 벡터
    edge1 = v2 - v1;
    edge2 = v3 - v2;
    edge3 = v1 - v3;

    % 점에서 각 변까지의 벡터
    c1 = points - v1; % 모든 점과 v1 간의 벡터
    c2 = points - v2; % 모든 점과 v2 간의 벡터
    c3 = points - v3; % 모든 점과 v3 간의 벡터

    % 외적 계산 (2D 외적은 z 성분만 사용)
    cross1 = edge1(1) * c1(:, 2) - edge1(2) * c1(:, 1);
    cross2 = edge2(1) * c2(:, 2) - edge2(2) * c2(:, 1);
    cross3 = edge3(1) * c3(:, 2) - edge3(2) * c3(:, 1);

    % 삼각형 내부 여부 판단 (외적의 부호가 모두 같아야 함)
    is_inside = (cross1 >= 0 & cross2 >= 0 & cross3 >= 0) | (cross1 <= 0 & cross2 <= 0 & cross3 <= 0);
end

== matlab function test_origin/Triggered Subsystem/계산 함수 ==
  data: K input; cameraPos input; cameraDir input; lightPos input; mesh input; beta input; C0 input; E_map output
function E_map = computeScatteringLighting(K, cameraPos, cameraDir, lightPos, mesh, beta, C0)
    % 입력:
    %   K: 3x3 Intrinsic Matrix (카메라 내부 파라미터 행렬)
    %   R_link: 3x3 Rotation Matrix (월드 좌표계 -> 링크 좌표계 회전 행렬)
    %   T: 3x1 Translation Vector (월드 좌표계 -> 링크 좌표계 이동 벡터)
    %   lightPos: 1x3 광원 위치 (월드 좌표계)
    %   mesh: 메쉬 데이터 (구조체)
    %       mesh.v:  정점(Vertices) 좌표 (Nx3 행렬, N: 정점 개수)
    %       mesh.f.v: 면(Faces)을 구성하는 정점 인덱스 (Mx3 행렬, M: 면 개수)
    %       mesh.f.vn: 면의 법선 벡터 (Mx3 행렬)
    %   beta: 감쇠 계수 (Attenuation Coefficient)
    %   C0: 광원의 초기 강도 (Initial Light Intensity)
    imageHeight = 480;
    imageWidth = 640;

    % 출력:
    %   E_map: imageHeight x imageWidth 크기의 2D 이미지. 각 픽셀은 해당 위치에 도달하는 빛의 에너지(세기)를 나타냄.

    % 1. 메쉬 데이터 가져오기
    vertices = mesh.vertices;      % 정점 좌표
    faces_vertex = mesh.faces.v; % 면을 구성하는 정점 인덱스
    normals = mesh.faces.vn;    % 면의 법선 벡터

    % 2. 출력 맵 초기화
    E_map = zeros(imageHeight, imageWidth); % 출력 이미지를 0으로 초기화
    numFaces = size(faces_vertex, 1);     % 면의 개수

    % 3. 월드 좌표계 -> 카메라 좌표계 변환 행렬 계산
    T_link = cameraPos; % 나중에 전치 주의!!

    quat_link_world = quaternion(cameraDir(1), cameraDir(2), cameraDir(3), cameraDir(4));
    R_w2link = rotmat(quat_link_world, 'frame')         % 월드 -> 링크 좌표계 회전
    R_link2cam =[0 -1 0; 0 0 -1; 1 0 0];                % 링크 좌표계 -> 카메라 좌표계 회전 
    
    Proj_w2link = [R_w2link, -R_w2link*T_link; 0,0,0,1];        % 동차 변환 행렬 (월드 -> 링크)
    Proj_link2Cam = [R_link2cam, zeros(3,1); zeros(1,3), 1];    % 동차 변환 행렬 (링크 -> 카메라)
    Proj_w2cam = Proj_link2Cam * Proj_w2link;                   % 동차 변환 행렬 (월드 -> 카메라)

    % 4. 광원 위치를 카메라 좌표계로 변환 (동차 좌표계 사용)
    lightPos_hom = [lightPos; 1]; % 광원 위치를 동차 좌표로
    lightPosCam_hom = Proj_w2cam * lightPos_hom;
    lightPosCam = lightPosCam_hom(1:3); % 다시 3차원 좌표로
    
   % 5. 각 면에 대해 반복
    for i = 1:numFaces
        % 5.1. 면의 세 정점 좌표 (월드 좌표계)
        v1 = vertices(faces_vertex(i, 1), :); % 첫 번째 정점
        v2 = vertices(faces_vertex(i, 2), :); % 두 번째 정점
        v3 = vertices(faces_vertex(i, 3), :); % 세 번째 정점

        % 5.2. 면 중심 (월드 좌표계)
        faceCenter = (v1 + v2 + v3) / 3;

        % 5.3. 면의 법선 벡터 (월드 좌표계, 정규화)
        normal = normals(i, :);
        normal = normal / norm(normal);

        % 5.4. 카메라 좌표계로 변환 (동차 좌표계 사용)
        faceCenter_hom = [faceCenter, 1]';
        faceCenterCam_hom = Proj_w2cam * faceCenter_hom;
        faceCenterCam = faceCenterCam_hom(1:3);

        v1_hom = [v1, 1]';
        v1_cam_hom = Proj_w2cam * v1_hom;
        v1_cam = v1_cam_hom(1:3);

        v2_hom = [v2, 1]';
        v2_cam_hom = Proj_w2cam * v2_hom;
        v2_cam = v2_cam_hom(1:3);

        v3_hom = [v3, 1]';
        v3_cam_hom = Proj_w2cam * v3_hom;
        v3_cam = v3_cam_hom(1:3);

        normal_hom = [normal, 0]'; % 방향 벡터는 마지막 요소가 0
        normalCam_hom = Proj_w2cam * normal_hom;
        normalCam = normalCam_hom(1:3);



        % 5.5. 광원 방향 (카메라 좌표계)
        lightDir = lightPosCam - faceCenterCam; % 면 중심 -> 광원
        lLS = norm(lightDir);              % 광원과 면 중심 사이의 거리
        lightDir = lightDir / lLS;           % 정규화

        % 5.6. Lambertian 반사 계수
        diffuseFactor = max(0, dot(normalCam, lightDir)); % (0 ~ 1)

        % 5.7. 직접광 (Ds) 계산
        Ds = (C0 * exp(-beta * lLS)) / (lLS^2);

        % 5.8. 산란 지점 (z) 계산 (카메라 좌표계)
        epsilon = 0.01; % 작은 값 (면에서 약간 떨어진 거리)
        z = faceCenterCam + epsilon * normalCam; % 면 중심에서 법선 방향으로

        % 5.9. 거리 계산 (카메라 좌표계)
        lLZ = norm(lightPosCam - z);     % 광원 -> 산란 지점
        lSZ = norm(z - faceCenterCam);   % 산란 지점 -> 면 중심
        lSC = norm(faceCenterCam);       % 면 중심 -> 카메라

        % 5.10. 산란광 (As) 계산
        As = (C0 * exp(-beta * (lLZ + lSZ))) / ((lLZ + lSZ)^2);

        % 5.11. 초기 조도, 최종 조도
        Es_initial = Ds + As;            % 직접광 + 산란광
        Es = Es_initial * exp(-beta * lSC); % 최종 감쇠

        % 5.12. 각 정점을 2D 이미지 좌표로 투영 (카메라 내부 파라미터 K 사용)
        v1_proj_hom = K * v1_cam;
        v1_proj = round(v1_proj_hom(1:2) / v1_proj_hom(3)); % 2D 픽셀 좌표

        v2_proj_hom = K * v2_cam;
        v2_proj = round(v2_proj_hom(1:2) / v2_proj_hom(3));

        v3_proj_hom = K * v3_cam;
        v3_proj = round(v3_proj_hom(1:2) / v3_proj_hom(3));


        % 5.13. 삼각형 래스터화 (Bresenham's Algorithm 기반)
        pixels = [];

        % 삼각형의 세 변을 따라 픽셀 좌표 생성
        pixels = [pixels; bresenham(v1_proj(1), v1_proj(2), v2_proj(1), v2_proj(2))];
        pixels = [pixels; bresenham(v2_proj(1), v2_proj(2), v3_proj(1), v3_proj(2))];
        pixels = [pixels; bresenham(v3_proj(1), v3_proj(2), v1_proj(1), v1_proj(2))];

        % 5.14. 삼각형 내부 픽셀에 대해 반복
        for p = 1:size(pixels, 1)
             x = pixels(p, 1); % 픽셀 x 좌표
             y = pixels(p, 2); % 픽셀 y 좌표

             % 픽셀이 이미지 범위 내에 있는지 확인
            if x < 1 || x > imageWidth || y < 1 || y > imageHeight
                continue;
            end

            % Barycentric Coordinates 계산
            [alpha, beta, gamma] = barycentric(x, y, v1_proj, v2_proj, v3_proj);

            if alpha >= 0 && beta >= 0 && gamma >= 0
                % 5.15. 픽셀 (x, y)에 E_s * diffuseFactor 값을 할당
                E_map(y, x) = Es * diffuseFactor;
            end
        end
    end % for i
end % function

% Bresenham's line algorithm 함수
function points = bresenham(x1, y1, x2, y2)
    % 입력: 두 점 (x1, y1), (x2, y2)
    % 출력: 두 점을 잇는 직선 상의 픽셀 좌표 (정수)

    points = [];
    dx = abs(x2 - x1);
    dy = abs(y2 - y1);
    sx = sign(x2 - x1);
    sy = sign(y2 - y1);
    err = dx - dy;

    x = x1;
    y = y1;

    while true
        points = [points; x, y];

        if x == x2 && y == y2
            break;
        end

        e2 = 2 * err;
        if e2 > -dy
            err = err - dy;
            x = x + sx;
        end
        if e2 < dx
            err = err + dx;
            y = y + sy;
        end
    end
end

% Barycentric coordinates 계산 함수
function [alpha, beta, gamma] = barycentric(x, y, v1, v2, v3)
    % 입력:
    %   x, y: 픽셀 좌표
    %   v1, v2, v3: 삼각형의 세 꼭지점 좌표 (2D)
    % 출력:
    %    alpha, beta, gamma: Barycentric Coordinates

    % 삼각형 면적 계산 (두 벡터의 외적)
    area = 0.5 * (-v2(2) * v3(1) + v1(2) * (-v2(1) + v3(1)) + v1(1) * (v2(2) - v3(2)) + v2(1) * v3(2));

    % 각 꼭지점에 대한 가중치 계산
    alpha = 0.5 * (-v2(2) * v3(1) + y * (-v2(1) + v3(1)) + x * (v2(2) - v3(2)) + v2(1) * v3(2)) / area;
    beta  = 0.5 * ( v1(2) * v3(1) - y * v3(1) + x * (-v1(2) + v3(2)) - v1(1) * v3(2)              ) / area;
    gamma = 0.5 * (-v1(2) * v2(1) + v1(2) * x + v2(2) * (-x + v1(1)) + y * (v2(1) - v1(1))) / area;

end

== matlab function test_origin/MATLAB Function2 ==
  data: u input; y output
function y = convertUInt8VarSizeToString(u)

y = convertCharsToStrings(char(u));

== matlab function test_origin/Triggered Subsystem/시각화 함수(물체, 카메라-조명) ==
  data: mesh input; cameraPos input; cameraDir input; lightPos input
function viz_scene(mesh, cameraPos, cameraDir, lightPos)

    persistent figHandle; % Figure 핸들을 저장할 persistent 변수

    if isempty(figHandle)
        % Figure가 없으면 (처음 실행) figHandle 초기화
        figHandle = figure;
        set(figHandle, 'Name', 'Scene Visualization'); % (선택 사항) 창 제목 설정
    elseif ~ishandle(figHandle) || ~strcmp(get(figHandle, 'Type'), 'figure')
        % Figure 핸들이 유효하지 않으면 (Figure가 닫힌 경우)
        figHandle = figure; % 새 Figure 생성
        set(figHandle, 'Name', 'Scene Visualization');
    end
    
    figure(figHandle); % 해당 Figure를 활성화
    clf;    % Figure 내용 clear  % clf(figHandle) 대신 clf 사용

    faces_vertex = mesh.faces.v;
    vertices = mesh.vertices;
    quat_link_world = quaternion(cameraDir(1), cameraDir(2), cameraDir(3), cameraDir(4));
    R_w2link = rotmat(quat_link_world, 'frame');         % 월드 -> 링크 좌표계 회전
    R_link2cam =[0 -1 0; 0 0 -1; 1 0 0];                % 링크 좌표계 -> 카메라 좌표계 회전


    % 1. 메쉬 그리기
    subplot(1, 2, 1); % 이 부분은 그대로 유지
    trisurf(faces_vertex, vertices(:,1), vertices(:,2), vertices(:,3), 'FaceColor', 'cyan', 'EdgeColor', 'k');
    hold on;
    % Face 중앙에 Face 번호 표시
    for i = 1:int32(size(faces_vertex, 1))
        % 현재 Face의 정점 3개 가져오기
        face_vertices = vertices(faces_vertex(i, :), :);

        % Face의 중심 좌표 계산
        face_center = mean(face_vertices, 1);

        % Face의 중앙에 번호 표시
        text(face_center(1), face_center(2), face_center(3), sprintf('%d',i), ...
            'FontSize', 12, 'FontWeight', 'bold', 'Color', 'r');
    end

    % 2. 카메라 위치 및 방향 (월드 좌표계)
    cameraPos_world = cameraPos; % 월드 좌표계에서의 카메라 위치
    R_world_to_cam = R_link2cam * R_w2link; % 카메라 방향 변환 행렬
    % 카메라 X축 (빨강)
    quiver3(cameraPos_world(1), cameraPos_world(2), cameraPos_world(3), ...
        R_world_to_cam(1,1), R_world_to_cam(2,1), R_world_to_cam(3,1), 0.3, 'r', 'LineWidth', 2, 'MaxHeadSize', 0.5);
    % 카메라 Y축 (초록)
    quiver3(cameraPos_world(1), cameraPos_world(2), cameraPos_world(3), ...
        R_world_to_cam(1,2), R_world_to_cam(2,2), R_world_to_cam(3,2), 0.3, 'g', 'LineWidth', 2, 'MaxHeadSize', 0.5);
    % 카메라 Z축 (파랑)
    quiver3(cameraPos_world(1), cameraPos_world(2), cameraPos_world(3), ...
        R_world_to_cam(1,3), R_world_to_cam(2,3), R_world_to_cam(3,3), 0.3, 'b', 'LineWidth', 2, 'MaxHeadSize', 0.5);

    % 카메라 위치 (빨간색 점)
    plot3(cameraPos_world(1), cameraPos_world(2), cameraPos_world(3), 'ro', 'MarkerSize', 8, 'MarkerFaceColor', 'r');
    % 3. 광원 위치
    plot3(lightPos(1), lightPos(2), lightPos(3), 'yo', 'MarkerSize', 10, 'MarkerFaceColor', 'y'); % 노란색 점
    % 축 및 레이블
    xlabel('X (World)');
    ylabel('Y (World)');
    zlabel('Z (World)');
    title('World Coordinate System (Mesh, Camera, Light)');
    axis equal;
    grid on;
    view(3);
    hold off;
end

== matlab function test_origin/Triggered Subsystem/시각화 함수(행렬) ==
  data: img input
function viz_mat(img)
    figure;
    imagesc(img);
    colorbar;
    title('E\_map (Scattering Lighting)');
    xlabel('Pixel X');
    ylabel('Pixel Y');
    axis image; % x, y 축 비율을 데이터에 맞게
end
